simulink model "case3_sim"  (R2023a)
settings: Solver=VariableStepAuto  StartTime=0.0  StopTime=10.0  RelTol=1e-3
values from neighbouring files (symbols this model uses):
  wn = 1/(R1*C1)    (= 1111.11111111)    [case3.m]
  zeta = ((R1*C1)+(R1*C2)+(R2*C2))/(2*wn*(R1*R2*C1*C2))    (= 1.5)    [case3.m]
settings Model: Creator=mazen  LastModifiedBy=mazen

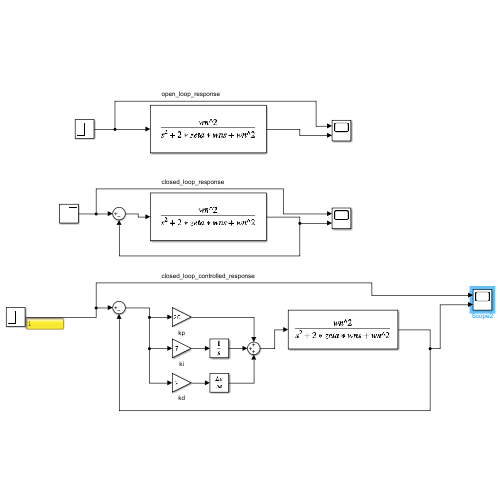
[thumbnail: Simulink's stored preview of the top-level diagram]
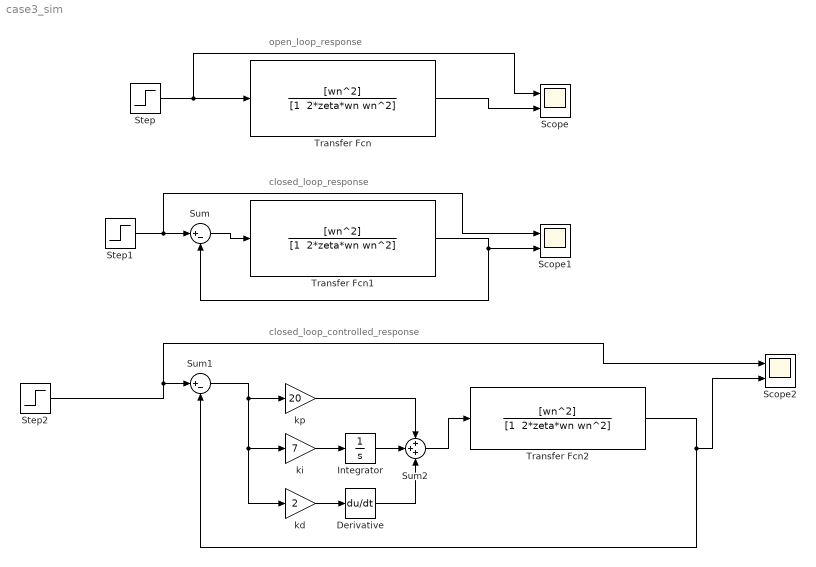
== system case3_sim ==
  note: closed_loop_response
  note: open_loop_response
  note: closed_loop_controlled_response
  Derivative : Derivative
  Integrator : Integrator
  Scope : Scope  NumInputPorts=2
  Scope1 : Scope  NumInputPorts=2
  Scope2 : Scope  NumInputPorts=2
  Step : Step  SampleTime=0
  Step1 : Step  SampleTime=0
  Step2 : Step  SampleTime=0
  Sum : Sum  Inputs=|+-
  Sum1 : Sum  Inputs=|+-
  Sum2 : Sum  Inputs=+++
  Transfer Fcn : TransferFcn  Numerator=[wn^2]  Denominator="[1  2*zeta*wn wn^2]"
  Transfer Fcn1 : TransferFcn  Numerator=[wn^2]  Denominator="[1  2*zeta*wn wn^2]"
  Transfer Fcn2 : TransferFcn  Numerator=[wn^2]  Denominator="[1  2*zeta*wn wn^2]"
  kd : Gain  Gain=2
  ki : Gain  Gain=7
  kp : Gain  Gain=20
  wires:
  ki/1 -> Integrator/1
  kp/1 -> Sum2/1
  Sum2/1 -> Transfer Fcn2/1
  kd/1 -> Derivative/1
  Sum/1 -> Transfer Fcn1/1
  Step1/1 -> Scope1/1, Sum/1
  Integrator/1 -> Sum2/2
  Transfer Fcn1/1 -> Scope1/2, Sum/2
  Transfer Fcn/1 -> Scope/2
  Derivative/1 -> Sum2/3
  Transfer Fcn2/1 -> Scope2/2, Sum1/2
  Sum1/1 -> kp/1, kd/1, ki/1
  Step/1 -> Scope/1, Transfer Fcn/1
  Step2/1 -> Scope2/1, Sum1/1
